simulink model "first_order_ADRC_MATLABfcn"  (R2017a)
settings: Solver=FixedStepAuto  StartTime=0.0  StopTime=10.0  FixedStep=0.0001  RelTol=1e-3
undefined symbols (not defined in the file or in its folder): b0, Kp
settings Model: Creator=rastronaut  LastModifiedBy=rastronaut

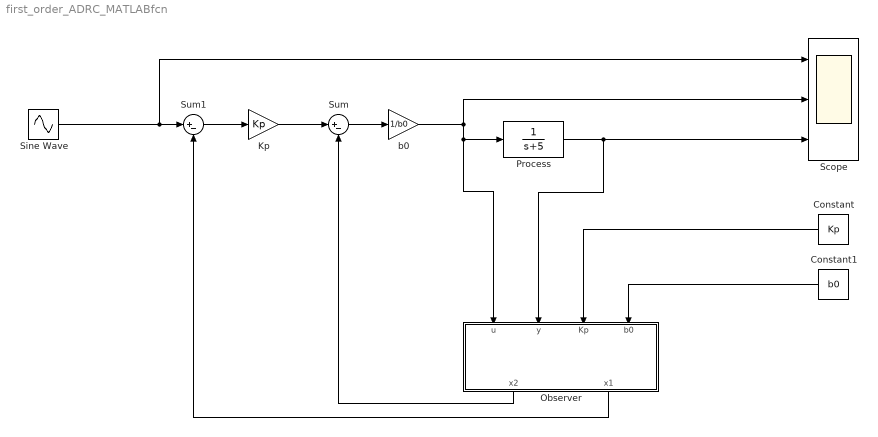
== system first_order_ADRC_MATLABfcn ==
  Constant : Constant  Value=Kp
  Constant1 : Constant  Value=b0
  Kp : Gain  Gain=Kp
  Observer : MATLAB Function  TreatAsAtomicUnit=on
  Process : TransferFcn  Denominator=[1 5]
  Scope : Scope  NumInputPorts=3
  Sine Wave : Sin  SampleTime=0
  Sum : Sum  Inputs=|+-
  Sum1 : Sum  Inputs=|+-
  b0 : Gain  Gain=1/b0
  wires:
  Kp/1 -> Sum/1
  Sum/1 -> b0/1
  Sum1/1 -> Kp/1
  b0/1 -> Observer/1(u), Process/1, Scope/2
  Process/1 -> Scope/3, Observer/2(y)
  Observer/1(x2) -> Sum/2
  Observer/2(x1) -> Sum1/2
  Sine Wave/1 -> Scope/1, Sum1/1
  Constant/1 -> Observer/3(Kp)
  Constant1/1 -> Observer/4(b0)

== matlab function first_order_ADRC_MATLABfcn/Observer ==
  data: x2 output; u input; x1 output; y input; Kp input; b0 input
function [x2, x1]= luenberger(u, y, Kp, b0)

persistent x1_old
persistent x2_old

if isempty(x1_old)
    x1_old = 0
end

if isempty(x2_old)
    x2_old = 0
end

Scl = -Kp;
Seso = 7*Scl;
l1 = -2*Seso;
l2 = Seso^2;

x1 = -l1*x1_old + b0*u + x2_old + l1*y
x2 = -l2*x1_old + l2*y;

x1_old = x1
x2_old = x2
